simulink model "part5"  (R2013a)
settings: Solver=ode45  StartTime=0.0  StopTime=t_end  RelTol=1e-7
values from neighbouring files (symbols this model uses):
  c = Beq + Bemf    (= 10.2235639816)    [lab1.m]
  gamma = (nu_g*Kg*nu_m*Kt)/(Rm*rmp)    (= 1.72354330709)    [lab1.m]
  kd = 20    [lab1.m]
  ki = 5    [lab1.m]
  kp = 400    [lab1.m]
  m = M + Mj    (= 1.07312664145)    [lab1.m]
libraries: simulink x2
settings Model: Creator=Willdog  LastModifiedBy=Willdog

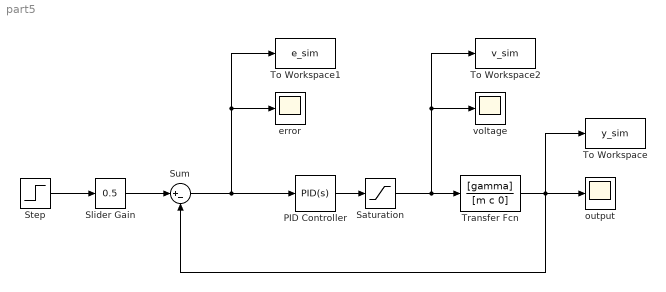
== system part5 ==
  PID Controller : simulink/Continuous/PID Controller  Controller=PID  TimeDomain=Continuous-time  SampleTime=1  IntegratorMethod=Forward Euler  FilterMethod=Forward Euler  Form=Parallel  P=kp  I=ki  D=kd  N=100  InitialConditionSource=internal  InitialConditionForIntegrator=0  InitialConditionForFilter=0  ExternalReset=none  LimitOutput=off  UpperSaturationLimit=inf  LowerSaturationLimit=-inf  LinearizeAsGain=on  AntiWindupMode=none  Kb=1  TrackingMode=off  Kt=1  PParamMin=[]  PParamMax=[]  IParamMin=[]  IParamMax=[]  DParamMin=[]  DParamMax=[]  NParamMin=[]  NParamMax=[]  KbParamMin=[]  KbParamMax=[]  KtParamMin=[]  KtParamMax=[]  POutMin=[]  POutMax=[]  IOutMin=[]  IOutMax=[]  DOutMin=[]  DOutMax=[]  NOutMin=[]  NOutMax=[]  KbOutMin=[]  KbOutMax=[]  KtOutMin=[]  KtOutMax=[]  IntegratorOutMin=[]  IntegratorOutMax=[]  FilterOutMin=[]  FilterOutMax=[]  SumOutMin=[]  SumOutMax=[]  SumI1OutMin=[]  SumI1OutMax=[]  SumI2OutMin=[]  SumI2OutMax=[]  SumI3OutMin=[]  SumI3OutMax=[]  SumDOutMin=[]  SumDOutMax=[]  SaturationOutMin=[]  SaturationOutMax=[]  IntegratorContinuousStateAttributes=''  IntegratorStateMustResolveToSignalObject=off  IntegratorRTWStateStorageClass=Auto  FilterContinuousStateAttributes=''  FilterStateMustResolveToSignalObject=off  FilterRTWStateStorageClass=Auto
  Saturation : Saturate  UpperLimit=6  LowerLimit=-6
  Slider Gain : simulink/Math Operations/Slider Gain  low=0  gain=0.5  high=2
  Step : Step  Time=0  SampleTime=0
  Sum : Sum  Inputs=|+-
  To Workspace : ToWorkspace  VariableName=y_sim  SampleTime=-1  SaveFormat=Timeseries
  To Workspace1 : ToWorkspace  VariableName=e_sim  SampleTime=-1  SaveFormat=Timeseries
  To Workspace2 : ToWorkspace  VariableName=v_sim  SampleTime=-1  SaveFormat=Timeseries
  Transfer Fcn : TransferFcn  Numerator=[gamma]  Denominator=[m c 0]
  error : Scope
  output : Scope
  voltage : Scope
      settings: SaveName=ScopeData2
  wires:
  Sum/1 -> To Workspace1/1, error/1, PID Controller/1
  Transfer Fcn/1 -> Sum/2, To Workspace/1, output/1
  PID Controller/1 -> Saturation/1
  Step/1 -> Slider Gain/1
  Slider Gain/1 -> Sum/1
  Saturation/1 -> voltage/1, To Workspace2/1, Transfer Fcn/1
